simulink model "quad_model_v4"  (R2026a)
settings: Solver=ode4  StopTime=20  FixedStep=0.01  RelTol=1e-6  AbsTol=1e-9
values from neighbouring files (symbols this model uses):
  g_acc = proj_params.g    [setup_quad_v4.m]
  mass = proj_params.m    [setup_quad_v4.m]
  motor_pwm_bp = (1000:10:2000)'    [setup_quad_v4.m]
  motor_Q_Nm = func_Q_lut(motor_pwm_bp)    [setup_quad_v4.m]
  motor_T_N = func_T_lut(motor_pwm_bp)    [setup_quad_v4.m]
  P_estimated = zeros(23,1)    [P_J_to_simulink.m]    (also in setup_quad_v4.m = P_J_to_simulink(P_J))
  phi0 = deg2rad(roll_deg(find(idx_w, 1, 'first')))    [setup_quad_v4.m]
  psi0 = deg2rad(yaw_deg(find(idx_w, 1, 'first')))    [setup_quad_v4.m]
  theta0 = deg2rad(pitch_deg(find(idx_w, 1, 'first')))    [setup_quad_v4.m]
undefined symbols (not defined in the file or in its folder): bias_acc, Lx_l, Lx_r, Ly_f, Ly_r, r_imu
libraries: matrix_library x1
settings Model: Creator=Henrique  LastModifiedBy=graest

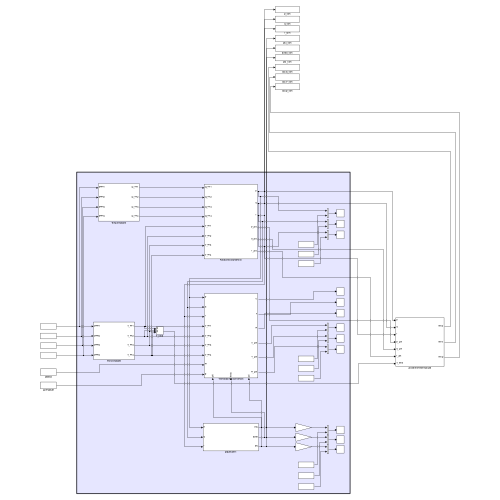
[thumbnail: Simulink's stored preview of the top-level diagram]
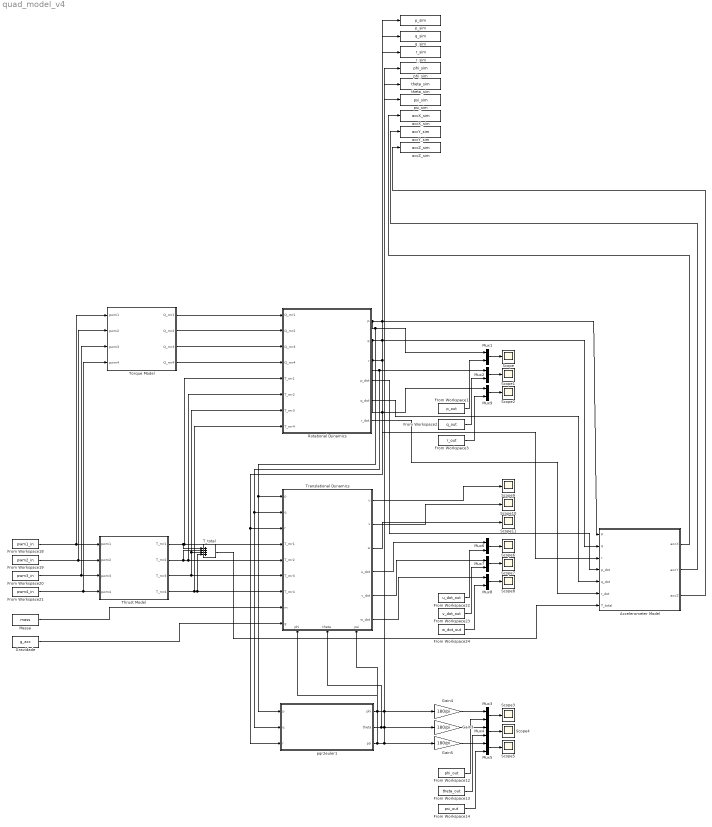
== system quad_model_v4 ==
  Accelerometer Model : Subsystem
  From Workspace1 : FromWorkspace  VariableName=p_out
  From Workspace12 : FromWorkspace  VariableName=phi_out
  From Workspace13 : FromWorkspace  VariableName=theta_out
  From Workspace14 : FromWorkspace  VariableName=psi_out
  From Workspace18 : FromWorkspace  VariableName=pwm1_in
  From Workspace19 : FromWorkspace  VariableName=pwm2_in
  From Workspace2 : FromWorkspace  VariableName=q_out
  From Workspace20 : FromWorkspace  VariableName=pwm3_in
  From Workspace21 : FromWorkspace  VariableName=pwm4_in
  From Workspace22 : FromWorkspace  VariableName=u_dot_out
  From Workspace23 : FromWorkspace  VariableName=v_dot_out
  From Workspace24 : FromWorkspace  VariableName=w_dot_out
  From Workspace3 : FromWorkspace  VariableName=r_out
  Gain3 : Gain  Gain=180/pi
  Gain4 : Gain  Gain=180/pi
  Gain5 : Gain  Gain=180/pi
  Gravidade : Constant  Value=g_acc
  Massa : Constant  Value=mass
  Mux{1..9} (9 alike) : Mux  Inputs=2
  Rotational Dynamics : Subsystem
  Scope{,1..11} (12 alike) : Scope
      Scope settings: ActiveDisplayYMinimum=-3.1838246882707533  ActiveDisplayYMaximum=2.3865969551138781  DataLoggingVariableName=ScopeData2
      Scope1 settings: ActiveDisplayYMinimum=-0.85222283188287973  ActiveDisplayYMaximum=0.80266881841056548  DataLoggingVariableName=ScopeData9
      Scope10 settings: ActiveDisplayYMinimum=-1  ActiveDisplayYMaximum=1  DataLoggingVariableName=ScopeData13
      Scope11 settings: ActiveDisplayYMinimum=-1  ActiveDisplayYMaximum=1  DataLoggingVariableName=ScopeData14
      Scope2 settings: ActiveDisplayYMinimum=-0.39909765778737721  ActiveDisplayYMaximum=0.46014245120214825  DataLoggingVariableName=ScopeData12
      Scope3 settings: ActiveDisplayYMinimum=-33.066128185692008  ActiveDisplayYMaximum=24.331982713695826  DataLoggingVariableName=ScopeData3
      Scope4 settings: ActiveDisplayYMinimum=-8.6113810330502787  ActiveDisplayYMaximum=8.1403061595645436  DataLoggingVariableName=ScopeData4
      Scope5 settings: ActiveDisplayYMinimum=161.43223403309159  ActiveDisplayYMaximum=201.61602542420681  DataLoggingVariableName=ScopeData5
      Scope6 settings: ActiveDisplayYMinimum=-1.3439733772979179  ActiveDisplayYMaximum=1.2986938828826189  DataLoggingVariableName=ScopeData6
      Scope7 settings: ActiveDisplayYMinimum=-2.4629833394773839  ActiveDisplayYMaximum=2.0408113951409432  DataLoggingVariableName=ScopeData7
      Scope8 settings: ActiveDisplayYMinimum=-12.400728468110792  ActiveDisplayYMaximum=-8.0186454243422123  DataLoggingVariableName=ScopeData8
      Scope9 settings: ActiveDisplayYMinimum=-0.55148333075895328  ActiveDisplayYMaximum=0.23226679011045651  DataLoggingVariableName=ScopeData15
  T_total : Sum  Inputs=++++
  Thrust Model : Subsystem
  Torque Model : Subsystem
  Translational Dynamics : Subsystem
      settings: PortSchema="{\"entries\":[{\"content\":{\"sides\":[{\"content\":{\"connectorIds\":[\"In1\",\"In2\",\"In3\",\"In4\",\"In5\",\"In6\",\"In7\",\"In8\",\"In9\"]},\"type\":\"ConnectorPlacement.EquallySpacedRectSide\",\"uuid\":\"f71b99dd-d086-42c5-ac61-061b6abdbb9c\"},{\"content\":{\"connectorIds\":[\"Out1\",\"Out2\",\"Out3\",\"Out4\",\"Out5\",\"Out6\"],\"side\":\"RIGHT\"},\"type\":\"ConnectorPlacement.EquallySpacedRectSide\",\"uuid\":\"0b5053fb-5501-424a-8925-f85dbe0224ed\"},{\"content\":{\"side\":\"TOP\"},\"type\":\"ConnectorPlacement.EquallySpacedRectSide\",\"uuid\":\"78179af8-06bb-410d-a49e-4acd134f9d12\"},{\"content\":{\"connectorIds\":[\"In10\",\"In11\",\"In12\"],\"side\":\"BOTTOM\"},\"type\":\"ConnectorPlacement.EquallySpacedRectSide\",\"uuid\":\"bdd8f061-0396-4374-a6c5-d0327680942c\"}]},\"type\":\"ConnectorPlacement.EquallySpacedConnector\",\"uuid\":\"f37cf57e-ef9d-4b35-a128-86db6ae39fb0\"}],\"packageUris\":[\"http://schema.mathworks.com/mf0/Connector/R2020b\"],\"version\":\"1.0\"}"
  accX_sim : ToWorkspace  VariableName=accX_sim  SaveFormat=Timeseries
  accY_sim : ToWorkspace  VariableName=accY_sim  SaveFormat=Timeseries
  accZ_sim : ToWorkspace  VariableName=accZ_sim  SaveFormat=Timeseries
  p_sim : ToWorkspace  VariableName=p_sim  SaveFormat=Timeseries
  phi_sim : ToWorkspace  VariableName=phi_sim  SaveFormat=Timeseries
  pqr2euler1 : Subsystem
  psi_sim : ToWorkspace  VariableName=psi_sim  SaveFormat=Timeseries
  q_sim : ToWorkspace  VariableName=q_sim  SaveFormat=Timeseries
  r_sim : ToWorkspace  VariableName=r_sim  SaveFormat=Timeseries
  theta_sim : ToWorkspace  VariableName=theta_sim  SaveFormat=Timeseries
  wires:
  Mux5/1 -> Scope5/1
  Mux3/1 -> Scope3/1
  From Workspace13/1 -> Mux4/2
  Gain5/1 -> Mux5/1
  From Workspace12/1 -> Mux3/2
  Gain4/1 -> Mux3/1
  pqr2euler1/1(phi) -> phi_sim/1, Gain4/1, Translational Dynamics/10(phi)
  Gain3/1 -> Mux4/1
  From Workspace14/1 -> Mux5/2
  pqr2euler1/2(theta) -> theta_sim/1, Gain3/1, Translational Dynamics/11(theta)
  Mux4/1 -> Scope4/1
  pqr2euler1/3(psi) -> psi_sim/1, Gain5/1, Translational Dynamics/12(psi)
  Mux7/1 -> Scope7/1
  Mux8/1 -> Scope8/1
  Mux6/1 -> Scope6/1
  From Workspace22/1 -> Mux6/2
  From Workspace23/1 -> Mux7/2
  From Workspace24/1 -> Mux8/2
  From Workspace19/1 -> Thrust Model/2(pwm2), Torque Model/2(pwm2)
  From Workspace20/1 -> Thrust Model/3(pwm3), Torque Model/3(pwm3)
  From Workspace21/1 -> Thrust Model/4(pwm4), Torque Model/4(pwm4)
  Thrust Model/1(T_mr1) -> Rotational Dynamics/5(T_mr1), Translational Dynamics/4(T_mr1), T_total/1
  Thrust Model/2(T_mr2) -> Rotational Dynamics/6(T_mr2), Translational Dynamics/5(T_mr2), T_total/2
  Thrust Model/3(T_mr3) -> T_total/3, Rotational Dynamics/7(T_mr3), Translational Dynamics/6(T_mr3)
  Thrust Model/4(T_mr4) -> T_total/4, Translational Dynamics/7(T_mr4), Rotational Dynamics/8(T_mr4)
  Massa/1 -> Translational Dynamics/8(m)
  Gravidade/1 -> Translational Dynamics/9(g)
  From Workspace18/1 -> Thrust Model/1(pwm1), Torque Model/1(pwm1)
  Torque Model/1(Q_mr1) -> Rotational Dynamics/1(Q_mr1)
  Torque Model/2(Q_mr2) -> Rotational Dynamics/2(Q_mr2)
  Torque Model/3(Q_mr3) -> Rotational Dynamics/3(Q_mr3)
  Torque Model/4(Q_mr4) -> Rotational Dynamics/4(Q_mr4)
  From Workspace2/1 -> Mux2/2
  Mux9/1 -> Scope2/1
  Rotational Dynamics/3(r) -> Accelerometer Model/3(r), r_sim/1, pqr2euler1/3(r), Translational Dynamics/3(r), Mux9/1
  Mux2/1 -> Scope1/1
  From Workspace1/1 -> Mux1/2
  From Workspace3/1 -> Mux9/2
  Mux1/1 -> Scope/1
  Rotational Dynamics/1(p) -> Accelerometer Model/1(p), p_sim/1, pqr2euler1/1(p), Translational Dynamics/1(p), Mux1/1
  Rotational Dynamics/2(q) -> Accelerometer Model/2(q), q_sim/1, pqr2euler1/2(q), Translational Dynamics/2(q), Mux2/1
  Translational Dynamics/4(u_dot) -> Mux6/1
  Translational Dynamics/5(v_dot) -> Mux7/1
  Translational Dynamics/6(w_dot) -> Mux8/1
  Translational Dynamics/1(u) -> Scope9/1
  Translational Dynamics/2(v) -> Scope10/1
  Translational Dynamics/3(w) -> Scope11/1
  Rotational Dynamics/4(p_dot) -> Accelerometer Model/4(p_dot)
  Rotational Dynamics/5(q_dot) -> Accelerometer Model/5(q_dot)
  Rotational Dynamics/6(r_dot) -> Accelerometer Model/6(r_dot)
  T_total/1 -> Accelerometer Model/7(T_total)
  Accelerometer Model/1(accX) -> accX_sim/1
  Accelerometer Model/2(accY) -> accY_sim/1
  Accelerometer Model/3(accZ) -> accZ_sim/1

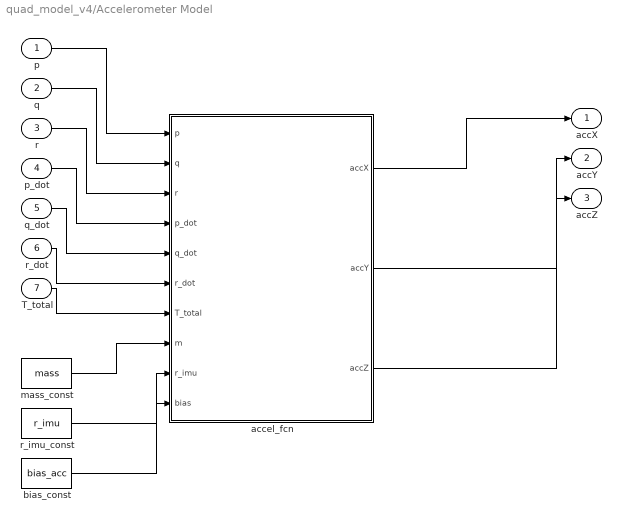
== system quad_model_v4/Accelerometer Model ==
  p : Inport
  q : Inport  Port=2
  r : Inport  Port=3
  p_dot : Inport  Port=4
  q_dot : Inport  Port=5
  r_dot : Inport  Port=6
  T_total : Inport  Port=7
  accel_fcn : MATLAB Function  TreatAsAtomicUnit=on
  bias_const : Constant  Value=bias_acc
  mass_const : Constant  Value=mass
  r_imu_const : Constant  Value=r_imu
  accX : Outport
  accY : Outport  Port=2
  accZ : Outport  Port=3
  wires:
  p/1 -> accel_fcn/1(p)
  q/1 -> accel_fcn/2(q)
  r/1 -> accel_fcn/3(r)
  p_dot/1 -> accel_fcn/4(p_dot)
  q_dot/1 -> accel_fcn/5(q_dot)
  r_dot/1 -> accel_fcn/6(r_dot)
  T_total/1 -> accel_fcn/7(T_total)
  mass_const/1 -> accel_fcn/8(m)
  r_imu_const/1 -> accel_fcn/9(r_imu)
  bias_const/1 -> accel_fcn/10(bias)
  accel_fcn/1(accX) -> accX/1
  accel_fcn/2(accY) -> accY/1
  accel_fcn/3(accZ) -> accZ/1

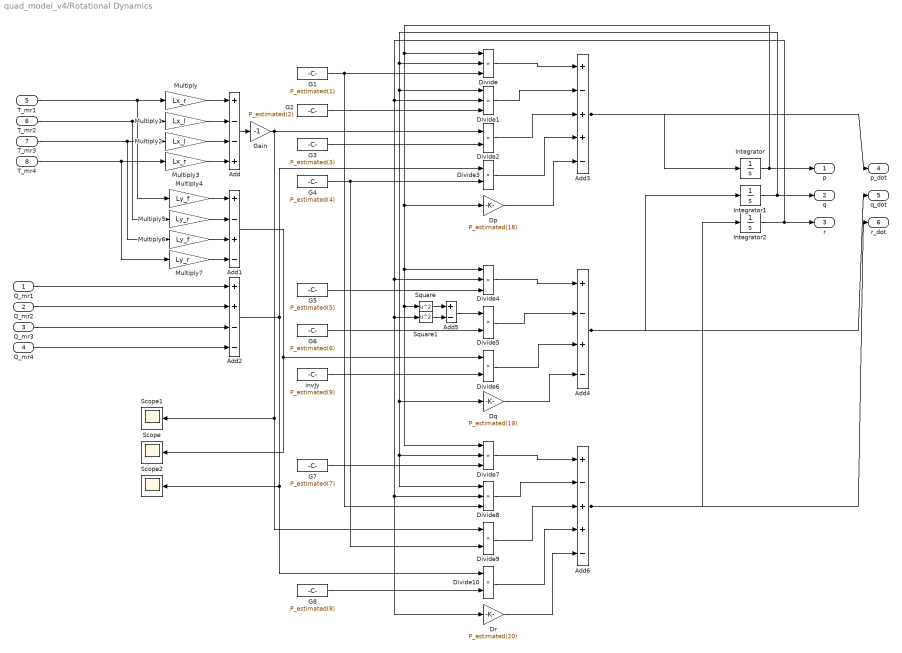
== system quad_model_v4/Rotational Dynamics ==
  Q_mr1 : Inport
  Q_mr2 : Inport  Port=2
  Q_mr3 : Inport  Port=3
  Q_mr4 : Inport  Port=4
  T_mr1 : Inport  Port=5
  T_mr2 : Inport  Port=6
  T_mr3 : Inport  Port=7
  T_mr4 : Inport  Port=8
  Add : Sum  Inputs=+--+
  Add1 : Sum  Inputs=+-+-
  Add2 : Sum  Inputs=++--
  Add3 : Sum  Inputs=+-++-
  Add4 : Sum  Inputs=+-+-
  Add5 : Sum  Inputs=+-
  Add6 : Sum  Inputs=+-++-
  Divide{,1,4,7..8} (5 alike) : Product  Inputs=***
  Divide{2..3,5..6,9..10} (6 alike) : Product  Inputs=**
  Dp : Gain  Gain=P_estimated(18)
  Dq : Gain  Gain=P_estimated(19)
  Dr : Gain  Gain=P_estimated(20)
  G1 : Constant  Value=P_estimated(1)
  G2 : Constant  Value=P_estimated(2)
  G3 : Constant  Value=P_estimated(3)
  G4 : Constant  Value=P_estimated(4)
  G5 : Constant  Value=P_estimated(5)
  G6 : Constant  Value=P_estimated(6)
  G7 : Constant  Value=P_estimated(7)
  G8 : Constant  Value=P_estimated(8)
  Gain : Gain  Gain=-1
  Integrator : Integrator
  Integrator1 : Integrator  InitialCondition=-0.1
  Integrator2 : Integrator  InitialCondition=-0.1
  Multiply : Gain  Gain=Lx_r
  Multiply1 : Gain  Gain=Lx_l
  Multiply2 : Gain  Gain=Lx_l
  Multiply3 : Gain  Gain=Lx_r
  Multiply4 : Gain  Gain=Ly_f
  Multiply5 : Gain  Gain=Ly_r
  Multiply6 : Gain  Gain=Ly_f
  Multiply7 : Gain  Gain=Ly_r
  Scope : Scope
      settings: ActiveDisplayYMinimum=-1.8186421464991014  ActiveDisplayYMaximum=1.3644776033104633
  Scope1 : Scope
      settings: ActiveDisplayYMinimum=-1.6294615313185898  ActiveDisplayYMaximum=1.5969792003618728  DataLoggingVariableName=ScopeData10
  Scope2 : Scope
      settings: ActiveDisplayYMinimum=-0.15040664283566432  ActiveDisplayYMaximum=0.048390422178986287  DataLoggingVariableName=ScopeData11
  Square : Math  Operator=square
  Square1 : Math  Operator=square
  invJy : Constant  Value=P_estimated(9)
  p : Outport
  q : Outport  Port=2
  r : Outport  Port=3
  p_dot : Outport  Port=4
  q_dot : Outport  Port=5
  r_dot : Outport  Port=6
  wires:
  Integrator/1 -> Divide4/1, Divide7/1, Square/1, Dp/1, Divide/1, p/1
  Integrator1/1 -> q/1, Divide8/1, Divide7/2, Dq/1, Divide1/1, Divide/2
  Integrator2/1 -> r/1, Divide4/2, Dr/1, Divide8/2, Square1/1, Divide1/2
  Multiply/1 -> Add/1
  Multiply1/1 -> Add/2
  Multiply2/1 -> Add/3
  Multiply3/1 -> Add/4
  T_mr2/1 -> Multiply5/1, Multiply1/1
  T_mr1/1 -> Multiply4/1, Multiply/1
  T_mr3/1 -> Multiply6/1, Multiply2/1
  T_mr4/1 -> Multiply7/1, Multiply3/1
  Q_mr1/1 -> Add2/1
  Q_mr2/1 -> Add2/2
  Q_mr3/1 -> Add2/3
  Q_mr4/1 -> Add2/4
  Multiply5/1 -> Add1/2
  Multiply7/1 -> Add1/4
  Multiply4/1 -> Add1/1
  Multiply6/1 -> Add1/3
  Add/1 -> Gain/1
  G1/1 -> Divide8/3, Divide/3
  G2/1 -> Divide1/3
  G3/1 -> Divide2/2
  Gain/1 -> Scope1/1, Divide9/1, Divide2/1
  G4/1 -> Divide9/2, Divide3/2
  Add2/1 -> Scope2/1, Divide10/1, Divide3/1
  Divide/1 -> Add3/1
  Divide1/1 -> Add3/2
  Divide2/1 -> Add3/3
  Divide3/1 -> Add3/4
  Dp/1 -> Add3/5
  Add3/1 -> Integrator/1, p_dot/1
  G5/1 -> Divide4/3
  Square/1 -> Add5/1
  Square1/1 -> Add5/2
  Divide4/1 -> Add4/1
  Add5/1 -> Divide5/1
  G6/1 -> Divide5/2
  invJy/1 -> Divide6/2
  Add1/1 -> Scope/1, Divide6/1
  Divide5/1 -> Add4/2
  Divide6/1 -> Add4/3
  Dq/1 -> Add4/4
  Add4/1 -> Integrator1/1, q_dot/1
  Divide7/1 -> Add6/1
  G7/1 -> Divide7/3
  Divide8/1 -> Add6/2
  G8/1 -> Divide10/2
  Divide9/1 -> Add6/3
  Divide10/1 -> Add6/4
  Dr/1 -> Add6/5
  Add6/1 -> Integrator2/1, r_dot/1

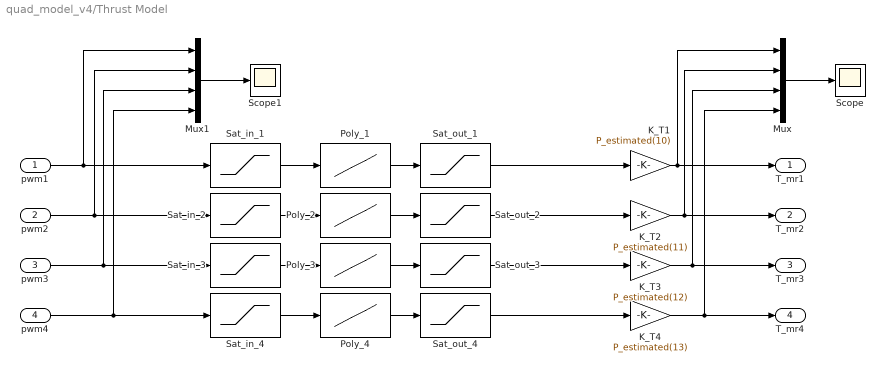
== system quad_model_v4/Thrust Model ==
  pwm1 : Inport
  pwm2 : Inport  Port=2
  pwm3 : Inport  Port=3
  pwm4 : Inport  Port=4
  K_T1 : Gain  Gain=P_estimated(10)
  K_T2 : Gain  Gain=P_estimated(11)
  K_T3 : Gain  Gain=P_estimated(12)
  K_T4 : Gain  Gain=P_estimated(13)
  Mux : Mux
  Mux1 : Mux
  Poly_{1..4} (4 alike) : Lookup_n-D  NumberOfTableDimensions=1  BreakpointsForDimension1=motor_pwm_bp  BreakpointsForDimension3=[5, 7]  Table=motor_T_N  InterpMethod=Akima spline  ExtrapMethod=Clip  InternalRulePriority=Speed  RndMeth=Simplest
  Sat_in_{1..4} (4 alike) : Saturate  UpperLimit=2000  LowerLimit=1000
  Sat_out_{1..4} (4 alike) : Saturate  UpperLimit=inf  LowerLimit=0
  Scope : Scope
      settings: ActiveDisplayYMinimum=-0.86498488922424888  ActiveDisplayYMaximum=7.4491008535267289
  Scope1 : Scope
      settings: ActiveDisplayYMinimum=1056.1863533445126  ActiveDisplayYMaximum=2048.2015162950543
  T_mr1 : Outport
  T_mr2 : Outport  Port=2
  T_mr3 : Outport  Port=3
  T_mr4 : Outport  Port=4
  wires:
  Mux/1 -> Scope/1
  Mux1/1 -> Scope1/1
  pwm2/1 -> Sat_in_2/1, Mux1/2
  pwm3/1 -> Sat_in_3/1, Mux1/3
  pwm1/1 -> Sat_in_1/1, Mux1/1
  pwm4/1 -> Sat_in_4/1, Mux1/4
  K_T1/1 -> Mux/1, T_mr1/1
  K_T2/1 -> Mux/2, T_mr2/1
  K_T3/1 -> Mux/3, T_mr3/1
  K_T4/1 -> Mux/4, T_mr4/1
  Sat_in_1/1 -> Poly_1/1
  Poly_1/1 -> Sat_out_1/1
  Sat_in_2/1 -> Poly_2/1
  Poly_2/1 -> Sat_out_2/1
  Sat_in_3/1 -> Poly_3/1
  Poly_3/1 -> Sat_out_3/1
  Sat_in_4/1 -> Poly_4/1
  Poly_4/1 -> Sat_out_4/1
  Sat_out_1/1 -> K_T1/1
  Sat_out_2/1 -> K_T2/1
  Sat_out_3/1 -> K_T3/1
  Sat_out_4/1 -> K_T4/1

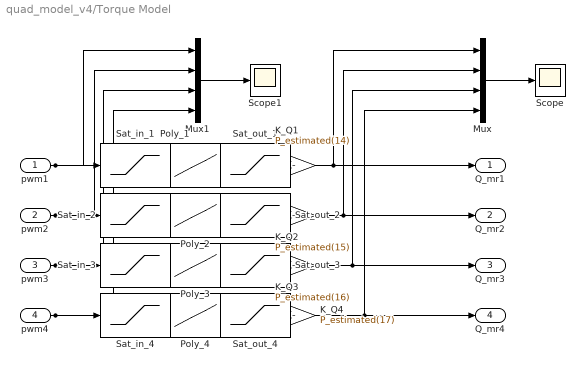
== system quad_model_v4/Torque Model ==
  pwm1 : Inport
  pwm2 : Inport  Port=2
  pwm3 : Inport  Port=3
  pwm4 : Inport  Port=4
  K_Q1 : Gain  Gain=P_estimated(14)
  K_Q2 : Gain  Gain=P_estimated(15)
  K_Q3 : Gain  Gain=P_estimated(16)
  K_Q4 : Gain  Gain=P_estimated(17)
  Mux : Mux
  Mux1 : Mux
  Poly_{1..4} (4 alike) : Lookup_n-D  NumberOfTableDimensions=1  BreakpointsForDimension1=motor_pwm_bp  BreakpointsForDimension3=[5, 7]  Table=motor_Q_Nm  InterpMethod=Akima spline  ExtrapMethod=Clip  InternalRulePriority=Speed  RndMeth=Simplest
  Sat_in_{1..4} (4 alike) : Saturate  UpperLimit=2000  LowerLimit=1000
  Sat_out_{1..4} (4 alike) : Saturate  UpperLimit=inf  LowerLimit=0
  Scope : Scope
      settings: ActiveDisplayYMinimum=-0.00070907967828830534  ActiveDisplayYMaximum=0.19742736062761823
  Scope1 : Scope
      settings: ActiveDisplayYMinimum=1056.1863533445126  ActiveDisplayYMaximum=2048.2015162950543
  Q_mr1 : Outport
  Q_mr2 : Outport  Port=2
  Q_mr3 : Outport  Port=3
  Q_mr4 : Outport  Port=4
  wires:
  Mux/1 -> Scope/1
  Mux1/1 -> Scope1/1
  pwm2/1 -> Mux1/2, Sat_in_2/1
  pwm3/1 -> Mux1/3, Sat_in_3/1
  pwm1/1 -> Mux1/1, Sat_in_1/1
  pwm4/1 -> Mux1/4, Sat_in_4/1
  K_Q1/1 -> Mux/1, Q_mr1/1
  K_Q2/1 -> Mux/2, Q_mr2/1
  K_Q3/1 -> Mux/3, Q_mr3/1
  K_Q4/1 -> Mux/4, Q_mr4/1
  Sat_in_1/1 -> Poly_1/1
  Poly_1/1 -> Sat_out_1/1
  Sat_in_2/1 -> Poly_2/1
  Poly_2/1 -> Sat_out_2/1
  Sat_in_3/1 -> Poly_3/1
  Poly_3/1 -> Sat_out_3/1
  Sat_in_4/1 -> Poly_4/1
  Poly_4/1 -> Sat_out_4/1
  Sat_out_1/1 -> K_Q1/1
  Sat_out_2/1 -> K_Q2/1
  Sat_out_3/1 -> K_Q3/1
  Sat_out_4/1 -> K_Q4/1

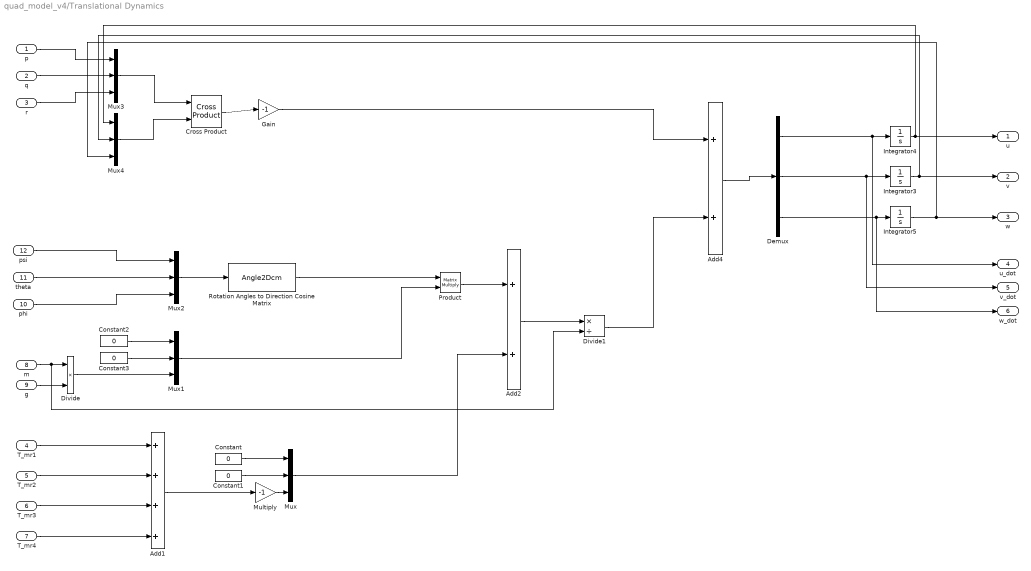
== system quad_model_v4/Translational Dynamics ==
  p : Inport
  q : Inport  Port=2
  r : Inport  Port=3
  T_mr1 : Inport  Port=4
  T_mr2 : Inport  Port=5
  T_mr3 : Inport  Port=6
  T_mr4 : Inport  Port=7
  m : Inport  Port=8
  g : Inport  Port=9
  phi : Inport  Port=10
  theta : Inport  Port=11
  psi : Inport  Port=12
  Add1 : Sum  Inputs=++++
  Add2 : Sum
  Add4 : Sum
  Constant{,1..3} (4 alike) : Constant  Value=0
  Cross Product : matrix_library/Cross Product
  Demux : Demux  Outputs=3
  Divide : Product  Inputs=**
  Divide1 : Product  Inputs=*/
  Gain : Gain  Gain=-1
  Integrator3 : Integrator
  Integrator4 : Integrator
  Integrator5 : Integrator
  Multiply : Gain  Gain=-1
  Mux{,1..4} (5 alike) : Mux  Inputs=3
  Product : Product  Multiplication=Matrix(*)
  Rotation Angles to Direction Cosine Matrix : Angle2Dcm
      settings: AttributesFormatString=Rotation Order: %<rotationOrder>
  u : Outport
  v : Outport  Port=2
  w : Outport  Port=3
  u_dot : Outport  Port=4
  v_dot : Outport  Port=5
  w_dot : Outport  Port=6
  wires:
  Multiply/1 -> Mux/3
  Add1/1 -> Multiply/1
  Constant/1 -> Mux/1
  Constant1/1 -> Mux/2
  T_mr4/1 -> Add1/4
  T_mr3/1 -> Add1/3
  T_mr2/1 -> Add1/2
  T_mr1/1 -> Add1/1
  Constant3/1 -> Mux1/2
  Constant2/1 -> Mux1/1
  Divide/1 -> Mux1/3
  m/1 -> Divide1/2, Divide/1
  g/1 -> Divide/2
  psi/1 -> Mux2/1
  theta/1 -> Mux2/2
  phi/1 -> Mux2/3
  Mux2/1 -> Rotation Angles to Direction Cosine Matrix/1
  Rotation Angles to Direction Cosine Matrix/1 -> Product/1
  Mux1/1 -> Product/2
  Product/1 -> Add2/1
  Mux/1 -> Add2/2
  p/1 -> Mux3/1
  q/1 -> Mux3/2
  r/1 -> Mux3/3
  Mux3/1 -> Cross Product/1
  Mux4/1 -> Cross Product/2
  Cross Product/1 -> Gain/1
  Add2/1 -> Divide1/1
  Gain/1 -> Add4/1
  Divide1/1 -> Add4/2
  Add4/1 -> Demux/1
  Demux/2 -> v_dot/1, Integrator3/1
  Demux/3 -> Integrator5/1, w_dot/1
  Demux/1 -> u_dot/1, Integrator4/1
  Integrator4/1 -> u/1, Mux4/1
  Integrator3/1 -> Mux4/2, v/1
  Integrator5/1 -> Mux4/3, w/1

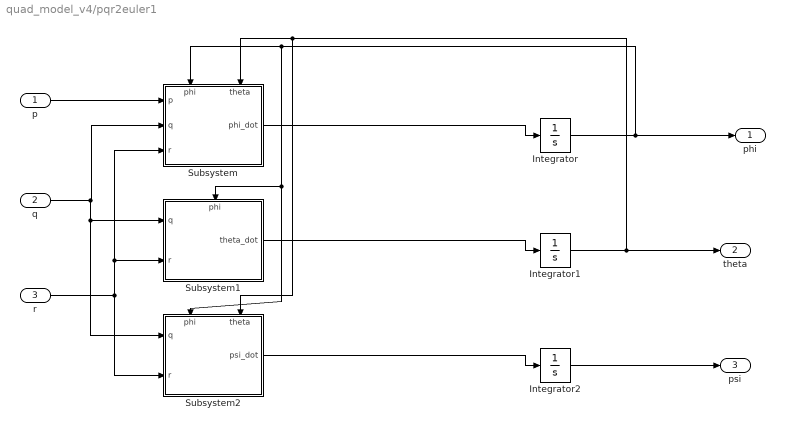
== system quad_model_v4/pqr2euler1 ==
  p : Inport
  q : Inport  Port=2
  r : Inport  Port=3
  Integrator : Integrator  InitialCondition=phi0
  Integrator1 : Integrator  InitialCondition=theta0
  Integrator2 : Integrator  InitialCondition=psi0
  Subsystem : Subsystem
      settings: PortSchema="{\"entries\":[{\"content\":{\"sides\":[{\"content\":{\"connectorIds\":[\"In1\",\"In2\",\"In3\"]},\"type\":\"ConnectorPlacement.EquallySpacedRectSide\",\"uuid\":\"382c9118-e079-49d8-ab8c-004ad07464e7\"},{\"content\":{\"connectorIds\":[\"Out1\"],\"side\":\"RIGHT\"},\"type\":\"ConnectorPlacement.EquallySpacedRectSide\",\"uuid\":\"72894542-f6bc-4d77-962a-2bf0bb014da1\"},{\"content\":{\"connectorIds\":[\"In4\",\"In5\"],\"side\":\"TOP\"},\"type\":\"ConnectorPlacement.EquallySpacedRectSide\",\"uuid\":\"7c36585a-f7f1-487a-9d1f-f469af8d2b77\"}]},\"type\":\"ConnectorPlacement.EquallySpacedConnector\",\"uuid\":\"a2cbdec5-7730-4b32-9373-0b6b5d68d7f2\"}],\"packageUris\":[\"http://schema.mathworks.com/mf0/Connector/R2020b\"],\"version\":\"1.0\"}"
  Subsystem1 : Subsystem
      settings: PortSchema="{\"entries\":[{\"content\":{\"sides\":[{\"content\":{\"connectorIds\":[\"In1\",\"In2\"]},\"type\":\"ConnectorPlacement.EquallySpacedRectSide\",\"uuid\":\"382c9118-e079-49d8-ab8c-004ad07464e7\"},{\"content\":{\"connectorIds\":[\"Out1\"],\"side\":\"RIGHT\"},\"type\":\"ConnectorPlacement.EquallySpacedRectSide\",\"uuid\":\"72894542-f6bc-4d77-962a-2bf0bb014da1\"},{\"content\":{\"connectorIds\":[\"In3\"],\"side\":\"TOP\"},\"type\":\"ConnectorPlacement.EquallySpacedRectSide\",\"uuid\":\"7c36585a-f7f1-487a-9d1f-f469af8d2b77\"}]},\"type\":\"ConnectorPlacement.EquallySpacedConnector\",\"uuid\":\"a2cbdec5-7730-4b32-9373-0b6b5d68d7f2\"}],\"packageUris\":[\"http://schema.mathworks.com/mf0/Connector/R2020b\"],\"version\":\"1.0\"}"
  Subsystem2 : Subsystem
      settings: PortSchema="{\"entries\":[{\"content\":{\"sides\":[{\"content\":{\"connectorIds\":[\"In1\",\"In2\"]},\"type\":\"ConnectorPlacement.EquallySpacedRectSide\",\"uuid\":\"382c9118-e079-49d8-ab8c-004ad07464e7\"},{\"content\":{\"connectorIds\":[\"Out1\"],\"side\":\"RIGHT\"},\"type\":\"ConnectorPlacement.EquallySpacedRectSide\",\"uuid\":\"72894542-f6bc-4d77-962a-2bf0bb014da1\"},{\"content\":{\"connectorIds\":[\"In3\",\"In4\"],\"side\":\"TOP\"},\"type\":\"ConnectorPlacement.EquallySpacedRectSide\",\"uuid\":\"7c36585a-f7f1-487a-9d1f-f469af8d2b77\"}]},\"type\":\"ConnectorPlacement.EquallySpacedConnector\",\"uuid\":\"a2cbdec5-7730-4b32-9373-0b6b5d68d7f2\"}],\"packageUris\":[\"http://schema.mathworks.com/mf0/Connector/R2020b\"],\"version\":\"1.0\"}"
  phi : Outport
  theta : Outport  Port=2
  psi : Outport  Port=3
  wires:
  Integrator/1 -> Subsystem2/3(phi), Subsystem1/3(phi), Subsystem/4(phi), phi/1
  Integrator1/1 -> Subsystem2/4(theta), Subsystem/5(theta), theta/1
  Integrator2/1 -> psi/1
  p/1 -> Subsystem/1(p)
  q/1 -> Subsystem2/1(q), Subsystem1/1(q), Subsystem/2(q)
  r/1 -> Subsystem2/2(r), Subsystem1/2(r), Subsystem/3(r)
  Subsystem/1(phi_dot) -> Integrator/1
  Subsystem1/1(theta_dot) -> Integrator1/1
  Subsystem2/1(psi_dot) -> Integrator2/1

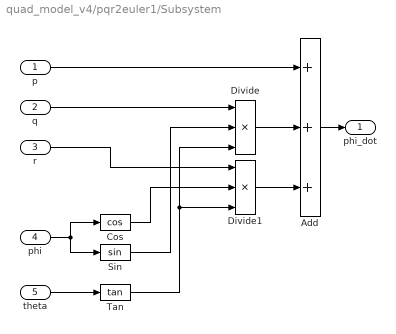
== system quad_model_v4/pqr2euler1/Subsystem ==
  p : Inport
  q : Inport  Port=2
  r : Inport  Port=3
  phi : Inport  Port=4
  theta : Inport  Port=5
  Add : Sum  Inputs=+++
  Cos : Trigonometry  Operator=cos
  Divide : Product  Inputs=***
  Divide1 : Product  Inputs=***
  Sin : Trigonometry
  Tan : Trigonometry  Operator=tan
  phi_dot : Outport
  wires:
  Add/1 -> phi_dot/1
  Divide1/1 -> Add/3
  Divide/1 -> Add/2
  p/1 -> Add/1
  phi/1 -> Sin/1, Cos/1
  theta/1 -> Tan/1
  q/1 -> Divide/1
  Sin/1 -> Divide/2
  Tan/1 -> Divide1/3, Divide/3
  r/1 -> Divide1/1
  Cos/1 -> Divide1/2

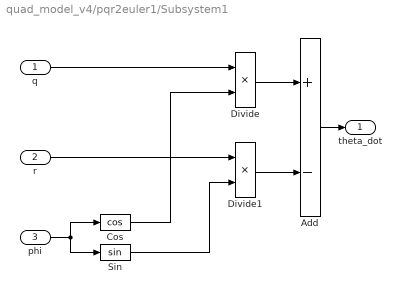
== system quad_model_v4/pqr2euler1/Subsystem1 ==
  q : Inport
  r : Inport  Port=2
  phi : Inport  Port=3
  Add : Sum  Inputs=+-
  Cos : Trigonometry  Operator=cos
  Divide : Product  Inputs=**
  Divide1 : Product  Inputs=**
  Sin : Trigonometry
  theta_dot : Outport
  wires:
  Add/1 -> theta_dot/1
  phi/1 -> Sin/1, Cos/1
  q/1 -> Divide/1
  r/1 -> Divide1/1
  Cos/1 -> Divide/2
  Sin/1 -> Divide1/2
  Divide/1 -> Add/1
  Divide1/1 -> Add/2

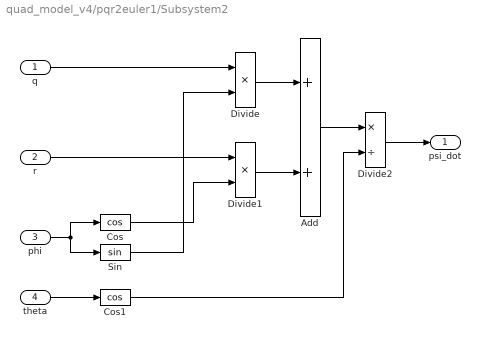
== system quad_model_v4/pqr2euler1/Subsystem2 ==
  q : Inport
  r : Inport  Port=2
  phi : Inport  Port=3
  theta : Inport  Port=4
  Add : Sum
  Cos : Trigonometry  Operator=cos
  Cos1 : Trigonometry  Operator=cos
  Divide : Product  Inputs=**
  Divide1 : Product  Inputs=**
  Divide2 : Product  Inputs=*/
  Sin : Trigonometry
  psi_dot : Outport
  wires:
  phi/1 -> Sin/1, Cos/1
  Divide/1 -> Add/1
  Divide1/1 -> Add/2
  theta/1 -> Cos1/1
  Add/1 -> Divide2/1
  Cos1/1 -> Divide2/2
  q/1 -> Divide/1
  Sin/1 -> Divide/2
  r/1 -> Divide1/1
  Cos/1 -> Divide1/2
  Divide2/1 -> psi_dot/1

== matlab function quad_model_v4/Accelerometer Model/accel_fcn ==
  data: p input size=1; accX output size=1; q input size=1; r input size=1; p_dot input size=1; q_dot input size=1; r_dot input size=1; T_total input size=1; m input size=1; r_imu input size=[3 1]; bias input size=[3 1]; accY output size=1; accZ output size=1
function [accX, accY, accZ] = fcn(p, q, r, p_dot, q_dot, r_dot, T_total, m, r_imu, bias)
%#codegen
% Replica accelerometer_model.m
%   f_imu = f_cg + alpha x r_imu + omega x (omega x r_imu) + bias
% Sem drag (Xu=Yv=Zw=0), so thrust em Z.

rx = r_imu(1); ry = r_imu(2); rz = r_imu(3);
T_m = T_total / m;

% Specific force no CG (sem drag - so thrust)
fz_cg = -T_m;

% Termo Euler: alpha x r_imu
eul_x = q_dot*rz - r_dot*ry;
eul_y = r_dot*rx - p_dot*rz;
eul_z = p_dot*ry - q_dot*rx;

% Termo centripeta: omega x (omega x r_imu)
cen_x = p*q*ry + p*r*rz - (q^2 + r^2)*rx;
cen_y = p*q*rx + q*r*rz - (p^2 + r^2)*ry;
cen_z = p*r*rx + q*r*ry - (p^2 + q^2)*rz;

accX = eul_x + cen_x + bias(1);
accY = eul_y + cen_y + bias(2);
accZ = fz_cg + eul_z + cen_z + bias(3);
end
